simulink model "PathCheck"  (R2018b)
settings: Solver=VariableStepAuto  StartTime=0.0  StopTime=10.0  RelTol=1e-3
undefined symbols (not defined in the file): checker_board, start_t, start_x, start_y
libraries: simulink x1, visionsources x1
settings Model: Creator=rittwik  LastModifiedBy=rittwik

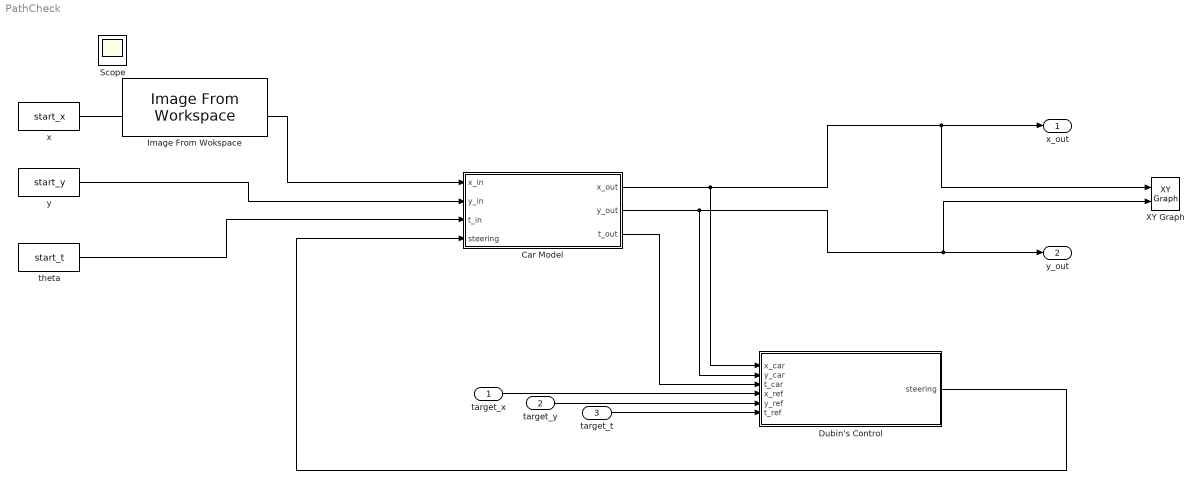
== system PathCheck ==
  target_x : Inport
  target_y : Inport  Port=2
  target_t : Inport  Port=3
  Car Model : Subsystem
  Dubin's Control : Subsystem
  XY Graph : simulink/Sinks/XY Graph  xmin=-1  xmax=1000  ymin=-1  ymax=1000  st=-1
  theta : Constant  Value=start_t
  x : Constant  Value=start_x
  y : Constant  Value=start_y
  x_out : Outport
  y_out : Outport  Port=2
  Image From Wokspace : visionsources/Image From Workspace  Tag=vipblks_nd  IOType=siggen  ImageValue=checker_board(10)  Ts=inf  imagePorts=One multidimensional signal  OutPortLabels=R|G|B  ImageDataType=Inherit from 'Value'  Signed=on  WordLength=16  sdImageDataType=sfix(16)  FractionLengthMode=User-defined  FractionLength=15
      settings: SourceProductName=Computer Vision System Toolbox  SourceProductBaseCode=VP
  Scope : Scope
  wires:
  x/1 -> Car Model/1(x_in)
  y/1 -> Car Model/2(y_in)
  theta/1 -> Car Model/3(t_in)
  Car Model/1(x_out) -> Dubin's Control/1(x_car), XY Graph/1, x_out/1
  Car Model/2(y_out) -> Dubin's Control/2(y_car), XY Graph/2, y_out/1
  Car Model/3(t_out) -> Dubin's Control/3(t_car)
  target_x/1 -> Dubin's Control/4(x_ref)
  target_y/1 -> Dubin's Control/5(y_ref)
  target_t/1 -> Dubin's Control/6(t_ref)
  Dubin's Control/1(steering) -> Car Model/4(steering)

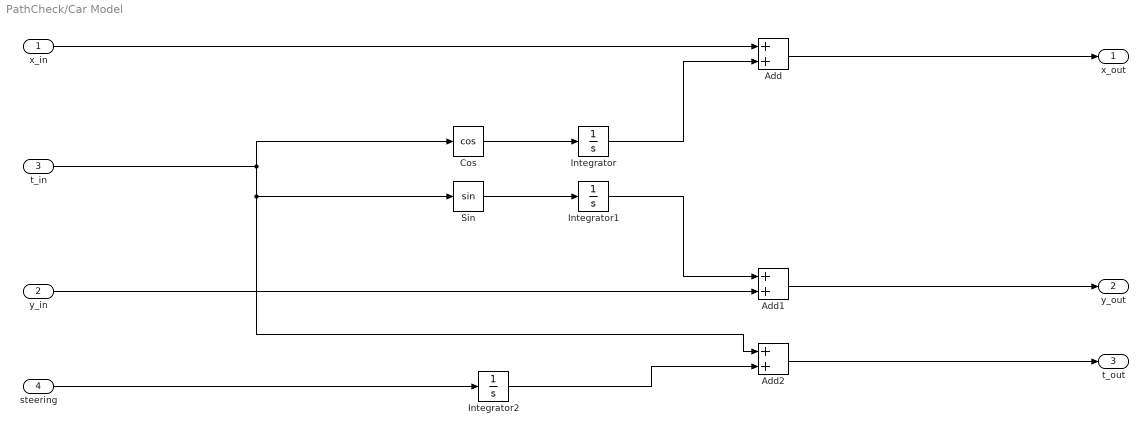
== system PathCheck/Car Model ==
  x_in : Inport
  y_in : Inport  Port=2
  t_in : Inport  Port=3
  steering : Inport  Port=4
  Add : Sum
  Add1 : Sum
  Add2 : Sum
  Cos : Trigonometry  Operator=cos
  Integrator : Integrator
  Integrator1 : Integrator
  Integrator2 : Integrator
  Sin : Trigonometry
  x_out : Outport
  y_out : Outport  Port=2
  t_out : Outport  Port=3
  wires:
  x_in/1 -> Add/1
  Add1/1 -> y_out/1
  Add/1 -> x_out/1
  Integrator/1 -> Add/2
  Cos/1 -> Integrator/1
  t_in/1 -> Cos/1, Add2/1, Sin/1
  Sin/1 -> Integrator1/1
  y_in/1 -> Add1/2
  Integrator1/1 -> Add1/1
  steering/1 -> Integrator2/1
  Integrator2/1 -> Add2/2
  Add2/1 -> t_out/1

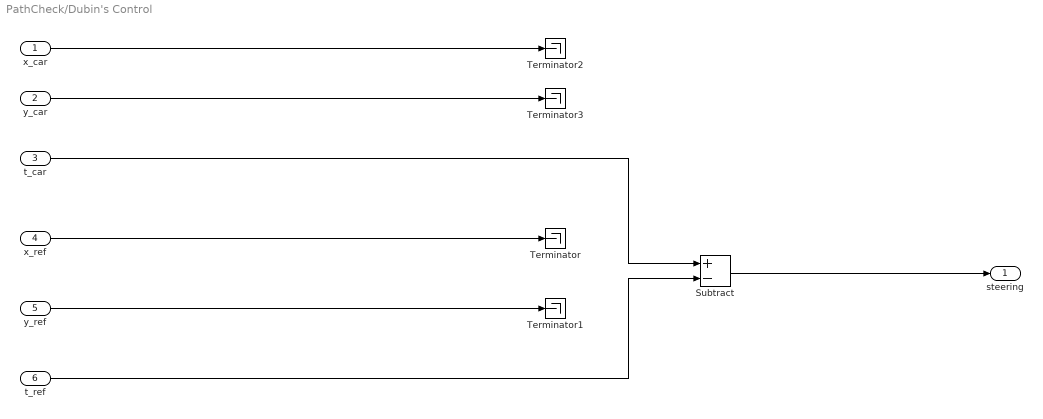
== system PathCheck/Dubin's Control ==
  x_car : Inport
  y_car : Inport  Port=2
  t_car : Inport  Port=3
  x_ref : Inport  Port=4
  y_ref : Inport  Port=5
  t_ref : Inport  Port=6
  Subtract : Sum  Inputs=+-
  Terminator{,1..3} (4 alike) : Terminator
  steering : Outport
  wires:
  t_car/1 -> Subtract/1
  t_ref/1 -> Subtract/2
  Subtract/1 -> steering/1
  y_ref/1 -> Terminator1/1
  x_car/1 -> Terminator2/1
  x_ref/1 -> Terminator/1
  y_car/1 -> Terminator3/1
